simulink model "walkgen"  (Simulink 7.0)
settings: Solver=FixedStepDiscrete  StartTime=0.0  StopTime=10  FixedStep=1e-3  RelTol=1e-3
libraries: simulink x7
Description:
  | Bringing in C++ Code into a C++ S-function Including Code Generation Support
CloseFcn:
  | rtwprivate ssgencode ModelCloseRequest walkgen
settings Model: Creator=The MathWorks Inc.  LastModifiedBy=herd_an  ExtModeTrigMode=oneshot  ExtModeArmWhenConnect=off  ExtModeAutoUpdateStatusClock=off
settings DataIOCC: LimitDataPoints=off  SaveOutput=off  SignalLogging=off  SaveTime=off  SignalLoggingName=logsOut
settings OptimizationCC: EnforceIntegerDowncast=off  StateBitsets=on  DataBitsets=on  UseTempVars=on  BufferReusableBoundary=off
settings DebuggingCC: SaveWithParameterizedLinksMsg=none  SignalResolutionControl=TryResolveAllWithWarning  SolverPrmCheckMsg=none  MultiTaskDSMMsg=warning  MultiTaskCondExecSysMsg=none  SigSpecEnsureSampleTimeMsg=none  StrictBusMsg=None
settings HardwareCC: ProdHWDeviceType=Specified  TargetHWDeviceType=32-bit Generic  ProdEqTarget=off
settings RTWCC: GenerateReport=on  RTWVerbose=off  ProcessScript=grt_make_rtw_hook  CustomSourceCode="#include \"sfun_cppcount_cpp.h\""  CustomInclude=../../../../simulink/src  CustomSource=sfun_cppcount_cpp.cpp  LaunchReport=on  TargetLang=C++  IncludeERTFirstTime=on
settings CodeAppCC: ForceParamTrailComments=on  CustomSymbolStrFcn=$F$N$M
settings GRTTargetCC: TargetFcnLib=ansi_tfl_tmw.mat

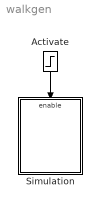
== system walkgen ==
  Activate : Step  Orientation=down  Time=0  SampleTime=0.001
  Simulation : Subsystem
  wires:
  Activate/1 -> Simulation/Enable

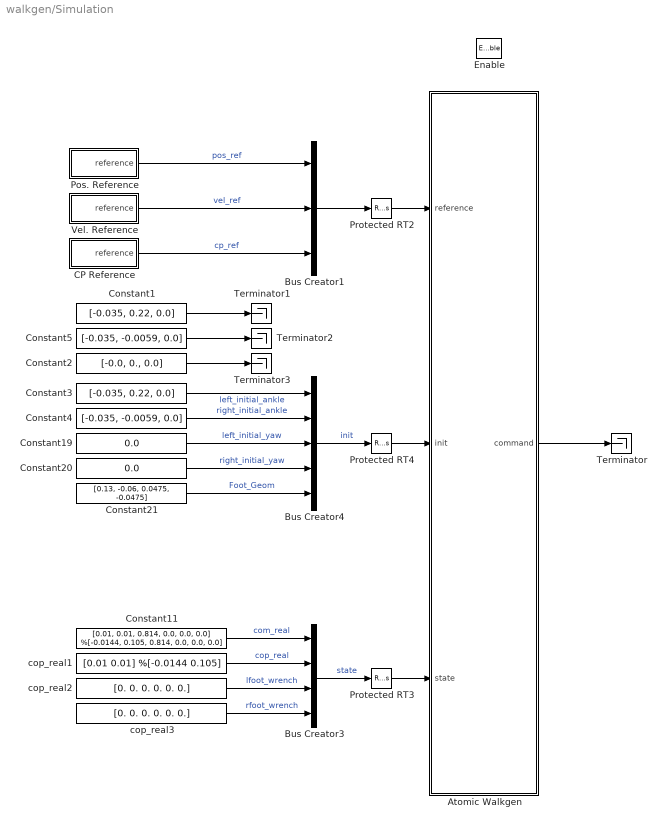
== system walkgen/Simulation ==
  Enable : EnablePort
  Atomic Walkgen : Subsystem  TreatAsAtomicUnit=on  SystemSampleTime=0.001  mask{num_samples_horizon=16, pos_weight=0, vel_weight=1, cop_weight=1, cp_weight=0, contr_moves_pen=0, first_contr_move_pen=0, num_samples_step=8, num_samples_dsss=8, num_steps_ssds=2, period_qpsample=0.1, period_mpcsample=0.1, period_actsample=0.001, security_margin=0.02, num_wsrec=100, dynamics_order=2, is_debug_mode=1, is_pid_mode=0, is_closed_loop=0, is_ineq_constraints=1, formulation=1, dump_problems=0, is_terminal_constr=0, solver=0, ds_force_thresh=100, ffoot_plan_period=1.6}
      mask prompts: num_samples_horizon "Length of horizon [num. samples]"; pos_weight "Position penalty"; vel_weight "Velocity penalty"; cop_weight "CoP penalty"; cp_weight "CP penalty"; contr_moves_pen "Control moves penalty"; first_contr_move_pen "First control move penalty"; num_samples_step "Step period [num. samples]"; num_samples_dsss "Length of initial double support phase [num. samples]"; num_steps_ssds "Steps before halt"; period_qpsample "Sampling period [s]"; period_mpcsample "Time between recomputations [s]"; period_actsample "Actuator sampling period [s]"; security_margin "Security margin [m]"; num_wsrec "Max number of working set recomputations"; dynamics_order "Dynamics order"; is_debug_mode "Debug mode"; is_pid_mode "PID mode"; is_closed_loop "Closed loop"; is_ineq_constraints "Inequality constraints"; formulation "Formulation (0 standard, 1 decoupled modes)"; dump_problems "Dump problems"; is_terminal_constr "Terminal constraints"; solver "Solver (0 QL, 1 QPOases, 2 LSSOL)"; ds_force_thresh "Force threshold for DS phase"; ffoot_plan_period "Foot placement planning period [s]"
  Bus Creator1 : BusCreator  Inputs=3
  Bus Creator3 : BusCreator
  Bus Creator4 : BusCreator  Inputs=5
  CP Reference : Subsystem
  Constant1 : Constant  Value=[-0.035, 0.22, 0.0]  OutDataType=sfix(16)  OutScaling=2^0
  Constant11 : Constant  Value=[0.01, 0.01, 0.814, 0.0, 0.0, 0.0] %[-0.0144, 0.105, 0.814, 0.0, 0.0, 0.0]  OutDataType=sfix(16)  OutScaling=2^0
  Constant19 : Constant  Value=0.0  OutDataType=sfix(16)  OutScaling=2^0
  Constant2 : Constant  Value=[-0.0, 0., 0.0]  OutDataType=sfix(16)  OutScaling=2^0
  Constant20 : Constant  Value=0.0  OutDataType=sfix(16)  OutScaling=2^0
  Constant21 : Constant  Value=[0.13, -0.06, 0.0475, -0.0475]  OutDataType=sfix(16)  OutScaling=2^0
  Constant3 : Constant  Value=[-0.035, 0.22, 0.0]  OutDataType=sfix(16)  OutScaling=2^0
  Constant4 : Constant  Value=[-0.035, -0.0059, 0.0]  OutDataType=sfix(16)  OutScaling=2^0
  Constant5 : Constant  Value=[-0.035, -0.0059, 0.0]  OutDataType=sfix(16)  OutScaling=2^0
  Pos. Reference : Subsystem
  Protected RT2 : RateTransition  Deterministic=off
  Protected RT3 : RateTransition  Deterministic=off
  Protected RT4 : RateTransition  Deterministic=off
  Terminator{,1..3} (4 alike) : Terminator
  Vel. Reference : Subsystem
  cop_real1 : Constant  Value=[0.01 0.01] %[-0.0144 0.105]  OutDataType=sfix(16)  OutScaling=2^0
  cop_real2 : Constant  Value=[0. 0. 0. 0. 0. 0.]  OutDataType=sfix(16)  OutScaling=2^0
  cop_real3 : Constant  Value=[0. 0. 0. 0. 0. 0.]  OutDataType=sfix(16)  OutScaling=2^0
  wires:
  Bus Creator3/1 -> Protected RT3/1  "state"
  Bus Creator4/1 -> Protected RT4/1  "init"
  Constant3/1 -> Bus Creator4/1  "left_initial_ankle"
  Constant4/1 -> Bus Creator4/2  "right_initial_ankle"
  Constant19/1 -> Bus Creator4/3  "left_initial_yaw"
  Constant20/1 -> Bus Creator4/4  "right_initial_yaw"
  Constant21/1 -> Bus Creator4/5  "Foot_Geom"
  Constant11/1 -> Bus Creator3/1  "com_real"
  cop_real1/1 -> Bus Creator3/2  "cop_real"
  Protected RT2/1 -> Atomic Walkgen/1(reference)
  Protected RT4/1 -> Atomic Walkgen/2(init)
  Protected RT3/1 -> Atomic Walkgen/3(state)
  Pos. Reference/1(reference) -> Bus Creator1/1  "pos_ref"
  Vel. Reference/1(reference) -> Bus Creator1/2  "vel_ref"
  CP Reference/1(reference) -> Bus Creator1/3  "cp_ref"
  Bus Creator1/1 -> Protected RT2/1
  Atomic Walkgen/1(command) -> Terminator/1
  cop_real2/1 -> Bus Creator3/3  "lfoot_wrench"
  cop_real3/1 -> Bus Creator3/4  "rfoot_wrench"
  Constant1/1 -> Terminator1/1
  Constant5/1 -> Terminator2/1
  Constant2/1 -> Terminator3/1

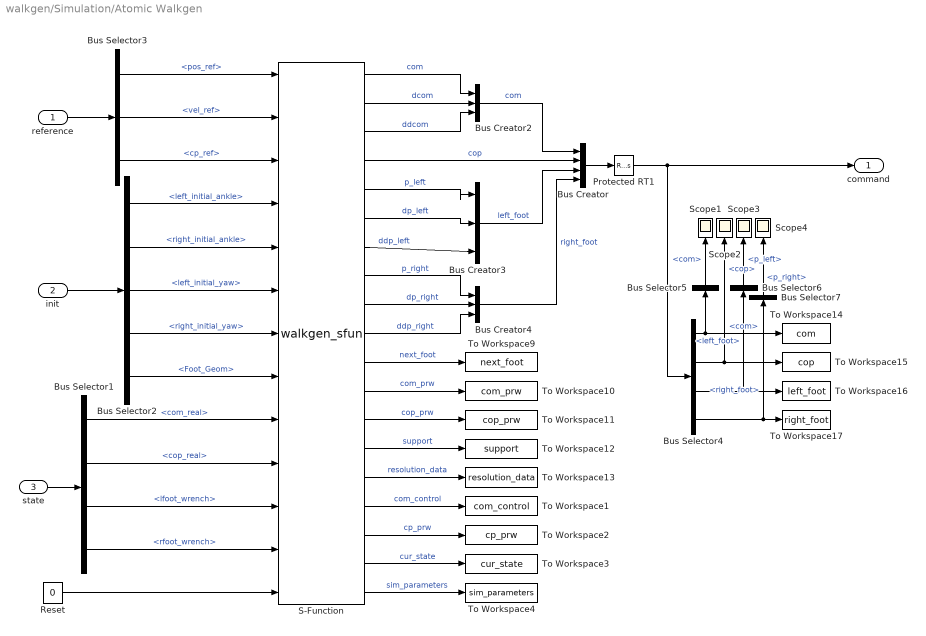
== system walkgen/Simulation/Atomic Walkgen ==
  reference : Inport  OutDataType=sfix(16)  OutScaling=2^0
  init : Inport  Port=2  OutDataType=sfix(16)  OutScaling=2^0
  state : Inport  Port=3  OutDataType=sfix(16)  OutScaling=2^0
  Bus Creator : BusCreator
  Bus Creator2 : BusCreator  Inputs=3
  Bus Creator3 : BusCreator  Inputs=3
  Bus Creator4 : BusCreator  Inputs=3
  Bus Selector1 : BusSelector  OutputSignals=com_real,cop_real,lfoot_wrench,rfoot_wrench
  Bus Selector2 : BusSelector  OutputSignals=left_initial_ankle,right_initial_ankle,left_initial_yaw,right_initial_yaw,Foot_Geom
  Bus Selector3 : BusSelector  OutputSignals=pos_ref,vel_ref,cp_ref
  Bus Selector4 : BusSelector  OutputSignals=com,cop,left_foot,right_foot
  Bus Selector5 : BusSelector  Orientation=up  OutputSignals=com
  Bus Selector6 : BusSelector  Orientation=up  OutputSignals=p_left
  Bus Selector7 : BusSelector  Orientation=up  OutputSignals=p_right
  Protected RT1 : RateTransition  Deterministic=off
  Reset : Constant  Value=0  OutDataType=sfix(16)  OutScaling=2^0
  S-Function : S-Function  FunctionName=walkgen_sfun  Parameters=num_samples_horizon, num_samples_step, num_samples_dsss, num_steps_ssds, period_qpsample, period_mpcsample, period_actsample, security_margin, num_wsrec, dynamics_order, is_debug_mode, pos_weight, vel_weight, cop_weight, cp_weight, contr_moves_pen, is_pid_mode, is_closed_loop, is_ineq_constraints, formulation, dump_problems, is_terminal_constr, solver, first_contr_move_pen, ds_force_thresh, ffoot_plan_period
  Scope{1..4} (4 alike) : Scope
      Scope1 settings: Orientation=up  TimeRange=3  YMin=-12  YMax=2
      Scope2 settings: Orientation=up  TimeRange=1  YMin=-0.1  YMax=0.25
      Scope3 settings: Orientation=up  TimeRange=0.5010330578512396  YMin=-1e-009  YMax=9e-009  SaveName=ScopeData2
      Scope4 settings: Orientation=up  TimeRange=0.5010330578512396  YMin=-1e-009  YMax=9e-009  SaveName=ScopeData3
  To Workspace1 : ToWorkspace  VariableName=com_control  SampleTime=-1  SaveFormat=Structure With Time
  To Workspace10 : ToWorkspace  VariableName=com_prw  SampleTime=-1  SaveFormat=Structure With Time
  To Workspace11 : ToWorkspace  VariableName=cop_prw  SampleTime=-1  SaveFormat=Structure With Time
  To Workspace12 : ToWorkspace  VariableName=support  SampleTime=-1  SaveFormat=Structure With Time
  To Workspace13 : ToWorkspace  VariableName=resolution_data  SampleTime=-1  SaveFormat=Structure With Time
  To Workspace14 : ToWorkspace  VariableName=com  SampleTime=-1  SaveFormat=Structure With Time
  To Workspace15 : ToWorkspace  VariableName=cop  SampleTime=-1  SaveFormat=Structure With Time
  To Workspace16 : ToWorkspace  VariableName=left_foot  SampleTime=-1  SaveFormat=Structure With Time
  To Workspace17 : ToWorkspace  VariableName=right_foot  SampleTime=-1  SaveFormat=Structure With Time
  To Workspace2 : ToWorkspace  VariableName=cp_prw  SampleTime=-1  SaveFormat=Structure With Time
  To Workspace3 : ToWorkspace  VariableName=cur_state  SampleTime=-1  SaveFormat=Structure With Time
  To Workspace4 : ToWorkspace  VariableName=sim_parameters  SampleTime=-1  SaveFormat=Structure With Time
  To Workspace9 : ToWorkspace  VariableName=next_foot  SampleTime=-1  SaveFormat=Structure With Time
  command : Outport  OutDataType=sfix(16)  OutScaling=2^0
  wires:
  Bus Creator/1 -> Protected RT1/1
  S-Function/1 -> Bus Creator2/1  "com"
  S-Function/4 -> Bus Creator/2  "cop"
  Bus Creator4/1 -> Bus Creator/4  "right_foot"
  S-Function/9 -> Bus Creator4/2  "dp_right"
  Bus Creator2/1 -> Bus Creator/1  "com"
  S-Function/2 -> Bus Creator2/2  "dcom"
  S-Function/3 -> Bus Creator2/3  "ddcom"
  Bus Creator3/1 -> Bus Creator/3  "left_foot"
  S-Function/10 -> Bus Creator4/3  "ddp_right"
  S-Function/5 -> Bus Creator3/1  "p_left"
  S-Function/6 -> Bus Creator3/2  "dp_left"
  S-Function/7 -> Bus Creator3/3  "ddp_left"
  S-Function/11 -> To Workspace9/1  "next_foot"
  S-Function/12 -> To Workspace10/1  "com_prw"
  S-Function/13 -> To Workspace11/1  "cop_prw"
  S-Function/14 -> To Workspace12/1  "support"
  S-Function/15 -> To Workspace13/1  "resolution_data"
  state/1 -> Bus Selector1/1
  init/1 -> Bus Selector2/1
  S-Function/16 -> To Workspace1/1  "com_control"
  S-Function/17 -> To Workspace2/1  "cp_prw"
  Protected RT1/1 -> command/1, Bus Selector4/1
  S-Function/8 -> Bus Creator4/1  "p_right"
  S-Function/18 -> To Workspace3/1  "cur_state"
  S-Function/19 -> To Workspace4/1  "sim_parameters"
  Bus Selector2/1 -> S-Function/4  "<left_initial_ankle>"
  Bus Selector2/2 -> S-Function/5  "<right_initial_ankle>"
  Bus Selector2/3 -> S-Function/6  "<left_initial_yaw>"
  Bus Selector2/4 -> S-Function/7  "<right_initial_yaw>"
  Bus Selector2/5 -> S-Function/8  "<Foot_Geom>"
  Bus Selector1/1 -> S-Function/9  "<com_real>"
  Bus Selector1/2 -> S-Function/10  "<cop_real>"
  reference/1 -> Bus Selector3/1
  Bus Selector3/1 -> S-Function/1  "<pos_ref>"
  Bus Selector3/2 -> S-Function/2  "<vel_ref>"
  Bus Selector3/3 -> S-Function/3  "<cp_ref>"
  Bus Selector4/1 -> To Workspace14/1, Bus Selector5/1  "<com>"
  Bus Selector4/2 -> To Workspace15/1, Scope2/1  "<cop>"
  Bus Selector4/3 -> To Workspace16/1, Bus Selector6/1  "<left_foot>"
  Bus Selector4/4 -> To Workspace17/1, Bus Selector7/1  "<right_foot>"
  Bus Selector5/1 -> Scope1/1  "<com>"
  Bus Selector6/1 -> Scope3/1  "<p_left>"
  Bus Selector7/1 -> Scope4/1  "<p_right>"
  Bus Selector1/3 -> S-Function/11  "<lfoot_wrench>"
  Bus Selector1/4 -> S-Function/12  "<rfoot_wrench>"
  Reset/1 -> S-Function/13

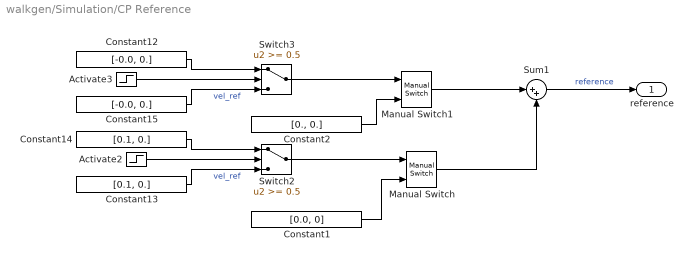
== system walkgen/Simulation/CP Reference ==
  Activate2 : Step  Time=10  SampleTime=0.001
  Activate3 : Step  Time=7  SampleTime=0.001
  Constant1 : Constant  Value=[0.0, 0]  OutDataType=sfix(16)  OutScaling=2^0
  Constant12 : Constant  Value=[-0.0, 0.]  OutDataType=sfix(16)  OutScaling=2^0
  Constant13 : Constant  Value=[0.1, 0.]  OutDataType=sfix(16)  OutScaling=2^0
  Constant14 : Constant  Value=[0.1, 0.]  OutDataType=sfix(16)  OutScaling=2^0
  Constant15 : Constant  Value=[-0.0, 0.]  OutDataType=sfix(16)  OutScaling=2^0
  Constant2 : Constant  Value=[0., 0.]  OutDataType=sfix(16)  OutScaling=2^0
  Manual Switch : simulink/Signal Routing/Manual Switch  SystemSampleTime=-1  sw=0  action=0  varsize=off
  Manual Switch1 : simulink/Signal Routing/Manual Switch  SystemSampleTime=-1  sw=0  action=0  varsize=off
  Sum1 : Sum  Inputs=|++  OutDataType=sfix(16)  OutScaling=2^0
  Switch2 : Switch  Threshold=0.5  OutDataType=sfix(16)  OutScaling=2^0
  Switch3 : Switch  Threshold=0.5  OutDataType=sfix(16)  OutScaling=2^0
  reference : Outport
  wires:
  Manual Switch1/1 -> Sum1/1
  Constant2/1 -> Manual Switch1/2
  Switch3/1 -> Manual Switch1/1
  Constant1/1 -> Manual Switch/2
  Manual Switch/1 -> Sum1/2
  Switch2/1 -> Manual Switch/1
  Sum1/1 -> reference/1  "reference"
  Activate3/1 -> Switch3/2
  Constant15/1 -> Switch3/3  "vel_ref"
  Constant12/1 -> Switch3/1
  Activate2/1 -> Switch2/2
  Constant13/1 -> Switch2/3  "vel_ref"
  Constant14/1 -> Switch2/1

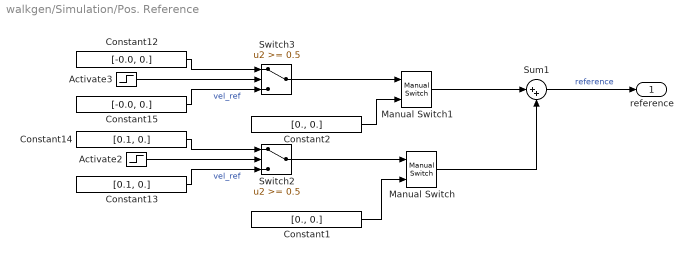
== system walkgen/Simulation/Pos. Reference ==
  Activate2 : Step  Time=10  SampleTime=0.001
  Activate3 : Step  Time=7  SampleTime=0.001
  Constant1 : Constant  Value=[0., 0.]  OutDataType=sfix(16)  OutScaling=2^0
  Constant12 : Constant  Value=[-0.0, 0.]  OutDataType=sfix(16)  OutScaling=2^0
  Constant13 : Constant  Value=[0.1, 0.]  OutDataType=sfix(16)  OutScaling=2^0
  Constant14 : Constant  Value=[0.1, 0.]  OutDataType=sfix(16)  OutScaling=2^0
  Constant15 : Constant  Value=[-0.0, 0.]  OutDataType=sfix(16)  OutScaling=2^0
  Constant2 : Constant  Value=[0., 0.]  OutDataType=sfix(16)  OutScaling=2^0
  Manual Switch : simulink/Signal Routing/Manual Switch  SystemSampleTime=-1  sw=0  action=0  varsize=off
  Manual Switch1 : simulink/Signal Routing/Manual Switch  SystemSampleTime=-1  sw=0  action=0  varsize=off
  Sum1 : Sum  Inputs=|++  OutDataType=sfix(16)  OutScaling=2^0
  Switch2 : Switch  Threshold=0.5  OutDataType=sfix(16)  OutScaling=2^0
  Switch3 : Switch  Threshold=0.5  OutDataType=sfix(16)  OutScaling=2^0
  reference : Outport
  wires:
  Manual Switch1/1 -> Sum1/1
  Constant2/1 -> Manual Switch1/2
  Switch3/1 -> Manual Switch1/1
  Constant1/1 -> Manual Switch/2
  Manual Switch/1 -> Sum1/2
  Switch2/1 -> Manual Switch/1
  Sum1/1 -> reference/1  "reference"
  Activate3/1 -> Switch3/2
  Constant15/1 -> Switch3/3  "vel_ref"
  Constant12/1 -> Switch3/1
  Activate2/1 -> Switch2/2
  Constant13/1 -> Switch2/3  "vel_ref"
  Constant14/1 -> Switch2/1

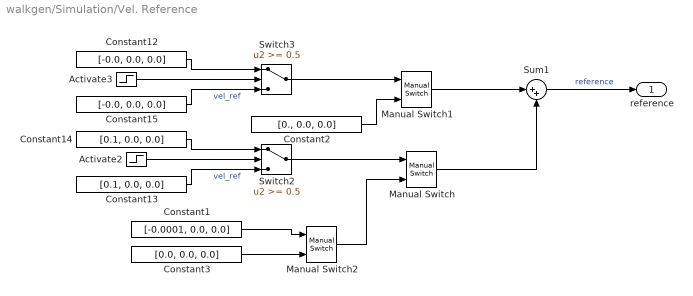
== system walkgen/Simulation/Vel. Reference ==
  Activate2 : Step  Time=10  SampleTime=0.001
  Activate3 : Step  Time=7  SampleTime=0.001
  Constant1 : Constant  Value=[-0.0001, 0.0, 0.0]  OutDataType=sfix(16)  OutScaling=2^0
  Constant12 : Constant  Value=[-0.0, 0.0, 0.0]  OutDataType=sfix(16)  OutScaling=2^0
  Constant13 : Constant  Value=[0.1, 0.0, 0.0]  OutDataType=sfix(16)  OutScaling=2^0
  Constant14 : Constant  Value=[0.1, 0.0, 0.0]  OutDataType=sfix(16)  OutScaling=2^0
  Constant15 : Constant  Value=[-0.0, 0.0, 0.0]  OutDataType=sfix(16)  OutScaling=2^0
  Constant2 : Constant  Value=[0., 0.0, 0.0]  OutDataType=sfix(16)  OutScaling=2^0
  Constant3 : Constant  Value=[0.0, 0.0, 0.0]  OutDataType=sfix(16)  OutScaling=2^0
  Manual Switch : simulink/Signal Routing/Manual Switch  SystemSampleTime=-1  sw=0  action=0  varsize=off
  Manual Switch1 : simulink/Signal Routing/Manual Switch  SystemSampleTime=-1  sw=0  action=0  varsize=off
  Manual Switch2 : simulink/Signal Routing/Manual Switch  SystemSampleTime=-1  sw=1  action=0  varsize=off
  Sum1 : Sum  Inputs=|++  OutDataType=sfix(16)  OutScaling=2^0
  Switch2 : Switch  Threshold=0.5  OutDataType=sfix(16)  OutScaling=2^0
  Switch3 : Switch  Threshold=0.5  OutDataType=sfix(16)  OutScaling=2^0
  reference : Outport
  wires:
  Constant14/1 -> Switch2/1
  Constant13/1 -> Switch2/3  "vel_ref"
  Activate2/1 -> Switch2/2
  Constant12/1 -> Switch3/1
  Constant15/1 -> Switch3/3  "vel_ref"
  Activate3/1 -> Switch3/2
  Sum1/1 -> reference/1  "reference"
  Switch2/1 -> Manual Switch/1
  Manual Switch/1 -> Sum1/2
  Switch3/1 -> Manual Switch1/1
  Constant2/1 -> Manual Switch1/2
  Manual Switch1/1 -> Sum1/1
  Constant1/1 -> Manual Switch2/1
  Constant3/1 -> Manual Switch2/2
  Manual Switch2/1 -> Manual Switch/2
